simulink model "Simulacion5_1_6_A"  (R2020a)
settings: Solver=VariableStepAuto  StartTime=0.0  StopTime=10.0  RelTol=1e-3
values from neighbouring files (symbols this model uses):
  alpha_cu = 3.9e-3    (= 0.0039)    [AnalisisDeEstabilidad.m]    (also in LTI_vs_LPV_vs_NL_realimentado.m; Modelo_linealizado.m; parametros.m)
  b_eq = b_m + b_l/(r^2)    (= 2.19444444444e-05)    [LTI_vs_LPV_vs_NL_realimentado.m]    (also in Modelo_linealizado.m; parametros.m)
  C_ts = 0.818    [LTI_vs_LPV_vs_NL_realimentado.m]    (also in Modelo_linealizado.m; parametros.m)
  J_eq = J_m + J_l/(r^2)    (= 1.97847222222e-05)    [LTI_vs_LPV_vs_NL_realimentado.m]    (also in Modelo_linealizado.m; parametros.m)
  L_d = 6.6/1000    (= 0.0066)    [Curvas_carc.m]    (also in LTI_vs_LPV_vs_NL_realimentado.m; Modelo_linealizado.m; parametros.m)
  L_ls = 0.8/1000    (= 0.0008)    [LTI_vs_LPV_vs_NL_realimentado.m]    (also in Modelo_linealizado.m; parametros.m)
  L_q = 5.8/1000    (= 0.0058)    [Curvas_carc.m]    (also in LTI_vs_LPV_vs_NL_realimentado.m; Modelo_linealizado.m; parametros.m)
  lambda_m = 0.01546    [Curvas_carc.m]    (also in LTI_vs_LPV_vs_NL_realimentado.m = 0.016; Modelo_linealizado.m = 0.016; parametros.m)
  P_p = 3    [Curvas_carc.m]    (also in LTI_vs_LPV_vs_NL_realimentado.m; parametros.m)
  Pp = 3    [AnalisisDeEstabilidad.m]    (also in LTI_vs_LPV_vs_NL_realimentado.m; Modelo_linealizado.m; parametros.m)
  r = 120    [AnalisisDeEstabilidad.m]    (also in LTI_vs_LPV_vs_NL_realimentado.m; Modelo_linealizado.m; parametros.m)
  R_s = 1.02    [Curvas_carc.m]    (also in LTI_vs_LPV_vs_NL_realimentado.m = R_s_o; Modelo_linealizado.m = 0.348; parametros.m)
  R_sREF = R_sref    (= 1.02)    [LTI_vs_LPV_vs_NL_realimentado.m]    (also in parametros.m)
  R_ts_amb = 146.7    [LTI_vs_LPV_vs_NL_realimentado.m]    (also in Modelo_linealizado.m; parametros.m)
  T_sREF = T_sref    (= 40)    [LTI_vs_LPV_vs_NL_realimentado.m]    (also in parametros.m)
undefined symbols (not defined in the file or in its folder): K_l
libraries: simulink x2
settings Model: Creator=matie  LastModifiedBy=matie

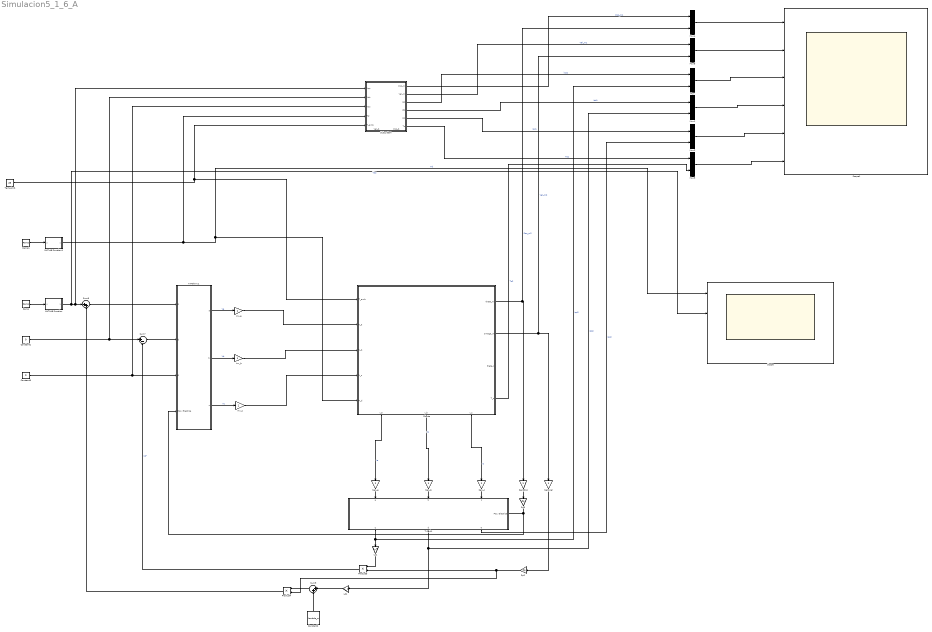
== system Simulacion5_1_6_A ==
  Constant1 : Constant  Value=0
  Constant2 : Constant  Value=lambda_m
  Constant3 : Constant  Value=0
  Inv_a : Gain
  Inv_b : Gain
  Inv_c : Gain
  Ld1 : Gain  Gain=L_d
  Lq1 : Gain  Gain=L_q
  MATLAB Function : MATLAB Function  TreatAsAtomicUnit=on
  MATLAB Function1 : MATLAB Function  TreatAsAtomicUnit=on
  Mux{,1..5} (6 alike) : Mux  Inputs=2
  Planta : Subsystem
      settings: PortSchema="{\"entries\":[{\"content\":{\"sides\":[{\"content\":{\"connectorIds\":[\"In1\",\"In2\",\"In3\",\"In4\",\"In5\"]},\"type\":\"ConnectorPlacement.EquallySpacedRectSide\",\"uuid\":\"7dd159b7-6d73-44ef-8a17-1619ab3a0fe8\"},{\"content\":{\"connectorIds\":[\"Out1\",\"Out2\",\"Out3\",\"Out4\"],\"side\":\"RIGHT\"},\"type\":\"ConnectorPlacement.EquallySpacedRectSide\",\"uuid\":\"f05f5aa2-2d36-48ca-b041-91fd4aa476a9\"},{\"content\":{\"connectorIds\":[],\"side\":\"TOP\"},\"type\":\"ConnectorPlacement.EquallySpacedRectSide\",\"uuid\":\"f00a682c-ef39-4c36-94cc-25936eb5c6a2\"},{\"content\":{\"connectorIds\":[\"Out5\",\"Out6\",\"Out7\"],\"side\":\"BOTTOM\"},\"type\":\"ConnectorPlacement.EquallySpacedRectSide\",\"uuid\":\"801a9ef0-d698-4696-ba24-5671b76f5cda\"}]},\"type\":\"ConnectorPlacement.EquallySpacedConnector\",\"uuid\":\"0722cfee-bb25-4366-9e08-c5916c966df5\"}],\"packageUris\":[\"http://schema.mathworks.com/mf0/Connector/19700101\"],\"version\":\"1.0\"}"
  Pp2 : Gain  Gain=Pp
  Pp3 : Gain  Gain=Pp
  Product3 : Product
  Product4 : Product
  Ramp : simulink/Sources/Ramp  slope=0  start=0  InitialOutput=0
  Ramp1 : simulink/Sources/Ramp  slope=1  start=0  InitialOutput=0
  Scope : Scope  NumInputPorts=4
  Scope1 : Scope  NumInputPorts=6
  Sen_Pos : Gain
  Sen_Vel : Gain
  Sen_a : Gain
  Sen_b : Gain
  Sen_c : Gain
  Subsystem : Subsystem
      settings: PortSchema="{\"entries\":[{\"content\":{\"sides\":[{\"content\":{\"connectorIds\":[\"In1\",\"In2\",\"In3\",\"In4\",\"In5\"]},\"type\":\"ConnectorPlacement.EquallySpacedRectSide\",\"uuid\":\"1d83102d-0bcd-437b-8c43-751b3339846b\"},{\"content\":{\"connectorIds\":[\"Out1\",\"Out2\",\"Out3\",\"Out4\",\"Out5\",\"Out6\"],\"side\":\"RIGHT\"},\"type\":\"ConnectorPlacement.EquallySpacedRectSide\",\"uuid\":\"75e93490-b52d-42b2-adb4-6c409fad0629\"},{\"content\":{\"connectorIds\":[],\"side\":\"TOP\"},\"type\":\"ConnectorPlacement.EquallySpacedRectSide\",\"uuid\":\"c21b1b05-3e78-438e-b61b-25f78d494297\"},{\"content\":{\"connectorIds\":[\"Out7\",\"Out8\"],\"side\":\"BOTTOM\"},\"type\":\"ConnectorPlacement.EquallySpacedRectSide\",\"uuid\":\"0978c98c-ad25-4e7d-b60c-0ad44d3b046e\"}]},\"type\":\"ConnectorPlacement.EquallySpacedConnector\",\"uuid\":\"d07407f3-9cdd-4509-bc17-68fd0115d69d\"}],\"packageUris\":[\"http://schema.mathworks.com/mf0/Connector/19700101\"],\"version\":\"1.0\"}"
  Sum7 : Sum  Inputs=|+-
  Sum8 : Sum  Inputs=|++
  Sum9 : Sum  Inputs=|++
  T.Park1 : Subsystem
      settings: PortSchema="{\"entries\":[{\"content\":{\"sides\":[{\"content\":{\"connectorIds\":[\"In1\",\"In2\",\"In3\"]},\"type\":\"ConnectorPlacement.EquallySpacedRectSide\",\"uuid\":\"2bfbe7ef-652a-4797-b13c-b84c243bd68c\"},{\"content\":{\"connectorIds\":[\"Out1\",\"Out2\",\"Out3\"],\"side\":\"RIGHT\"},\"type\":\"ConnectorPlacement.EquallySpacedRectSide\",\"uuid\":\"075def0e-c436-44dc-ba25-82cf6ffae869\"},{\"content\":{\"connectorIds\":[],\"side\":\"TOP\"},\"type\":\"ConnectorPlacement.EquallySpacedRectSide\",\"uuid\":\"95d81334-e332-4f04-a2cb-c4692f91809c\"},{\"content\":{\"connectorIds\":[\"In4\"],\"side\":\"BOTTOM\"},\"type\":\"ConnectorPlacement.EquallySpacedRectSide\",\"uuid\":\"85b95360-e43d-49d1-a18f-690334b045e6\"}]},\"type\":\"ConnectorPlacement.EquallySpacedConnector\",\"uuid\":\"b90f9cad-0277-459c-bcac-17172872a787\"}],\"packageUris\":[\"http://schema.mathworks.com/mf0/Connector/19700101\"],\"version\":\"1.0\"}"
  T.ParkInv1 : Subsystem
  TempAmb : Constant  Value=25
  wires:
  Constant3/1 -> Subsystem/3(Vos), T.ParkInv1/3(0)
  Sen_c/1 -> T.Park1/3(c)
  Constant1/1 -> Subsystem/2(Vds), Sum7/1
  Sum7/1 -> T.ParkInv1/2(d)
  T.ParkInv1/1(a) -> Inv_a/1  "Va"
  MATLAB Function/1(y) -> Scope/2, Subsystem/1(Vqs), Sum8/1  "Vqs"
  T.ParkInv1/2(b) -> Inv_b/1  "Vb"
  T.ParkInv1/3(c) -> Inv_c/1  "Vc"
  Ramp/1 -> MATLAB Function/1(u)
  Ramp1/1 -> MATLAB Function1/1(u)
  Sum8/1 -> T.ParkInv1/1(q)
  Sum9/1 -> Product4/1
  Product4/1 -> Sum8/2
  Sen_a/1 -> T.Park1/1(a)
  T.Park1/2(d) -> Mux1/2, Ld1/1  "ids2"
  Ld1/1 -> Sum9/1
  T.Park1/1(q) -> Lq1/1, Mux/2  "iqs2"
  Constant2/1 -> Sum9/2
  Sen_Pos/1 -> Pp3/1
  Planta/6(I_b) -> Sen_b/1  "Ib"
  Inv_c/1 -> Planta/4(V_c)
  Sen_b/1 -> T.Park1/2(b)
  MATLAB Function1/1(y) -> Subsystem/4(Td), Planta/5(T_d), Scope/1  "Td"
  Inv_a/1 -> Planta/2(V_a)
  Pp2/1 -> Product4/2, Product3/2
  Planta/5(I_a) -> Sen_a/1  "Ia"
  Sen_Vel/1 -> Pp2/1
  Planta/7(I_c) -> Sen_c/1  "Ic"
  Inv_b/1 -> Planta/3(V_b)
  TempAmb/1 -> Planta/1(T_amb), Subsystem/5(T_amb)
  Pp3/1 -> T.ParkInv1/4(Pos. Electrica), T.Park1/4(Pos. Electrica)
  Lq1/1 -> Product3/1
  Product3/1 -> Sum7/2  "Vd*"
  Subsystem/1(Pos_m) -> Mux4/1  "Pos_m1"
  Subsystem/2(Vel_m) -> Mux5/1  "Vel_m1"
  Subsystem/3(iqs) -> Mux/1  "iqs1"
  Subsystem/4(ids) -> Mux1/1  "ids1"
  Subsystem/5(ios) -> Mux2/1  "ios1"
  Subsystem/6(Ts) -> Mux3/1  "Ts1"
  Planta/2(omega_m) -> Mux5/2, Sen_Vel/1  "Vel_m2"
  Planta/1(theta_m) -> Mux4/2, Sen_Pos/1  "Pos_m2"
  T.Park1/3(0) -> Mux2/2  "ios2"
  Planta/4(T_s) -> Mux3/2  "Ts2"
  Mux4/1 -> Scope1/1
  Mux5/1 -> Scope1/2
  Mux/1 -> Scope1/3
  Mux1/1 -> Scope1/4
  Mux2/1 -> Scope1/5
  Mux3/1 -> Scope1/6

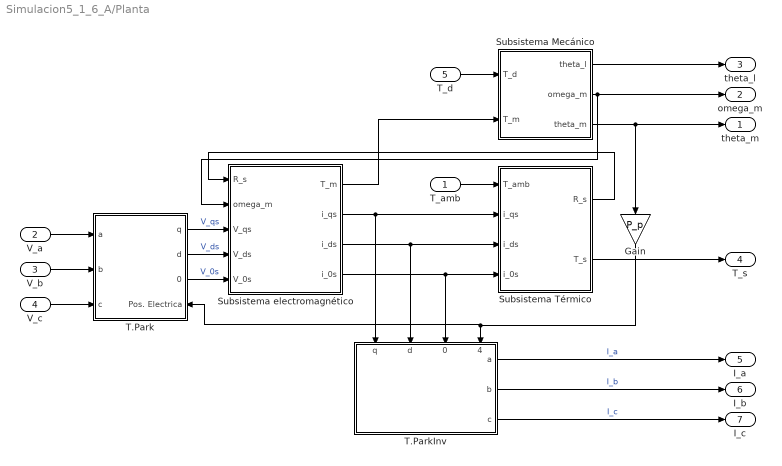
== system Simulacion5_1_6_A/Planta ==
  T_amb : Inport
  V_a : Inport  Port=2
  V_b : Inport  Port=3
  V_c : Inport  Port=4
  T_d : Inport  Port=5
  "\tSubsistema Térmico" : Subsystem
  Gain : Gain  Gain=P_p
  Subsistema Mecánico : Subsystem
  Subsistema electromagnético : Subsystem
  T.Park : Subsystem
      settings: PortSchema="{\"entries\":[{\"content\":{\"sides\":[{\"content\":{\"connectorIds\":[\"In1\",\"In2\",\"In3\"]},\"type\":\"ConnectorPlacement.EquallySpacedRectSide\",\"uuid\":\"2bfbe7ef-652a-4797-b13c-b84c243bd68c\"},{\"content\":{\"connectorIds\":[\"Out1\",\"Out2\",\"Out3\",\"In4\"],\"side\":\"RIGHT\"},\"type\":\"ConnectorPlacement.EquallySpacedRectSide\",\"uuid\":\"075def0e-c436-44dc-ba25-82cf6ffae869\"},{\"content\":{\"connectorIds\":[],\"side\":\"TOP\"},\"type\":\"ConnectorPlacement.EquallySpacedRectSide\",\"uuid\":\"95d81334-e332-4f04-a2cb-c4692f91809c\"}]},\"type\":\"ConnectorPlacement.EquallySpacedConnector\",\"uuid\":\"b90f9cad-0277-459c-bcac-17172872a787\"}],\"packageUris\":[\"http://schema.mathworks.com/mf0/Connector/19700101\"],\"version\":\"1.0\"}"
  T.ParkInv : Subsystem
      settings: PortSchema="{\"entries\":[{\"content\":{\"sides\":[{\"content\":{\"connectorIds\":[\"In1\",\"In2\",\"In3\",\"In4\"]},\"type\":\"ConnectorPlacement.EquallySpacedRectSide\",\"uuid\":\"aef3590a-5fc0-4a95-8f41-1fc79c0f3fe7\"},{\"content\":{\"connectorIds\":[],\"side\":\"RIGHT\"},\"type\":\"ConnectorPlacement.EquallySpacedRectSide\",\"uuid\":\"4e7c387b-9bca-48cc-a151-2357bd6b7b1d\"},{\"content\":{\"connectorIds\":[],\"side\":\"TOP\"},\"type\":\"ConnectorPlacement.EquallySpacedRectSide\",\"uuid\":\"1231932f-f9d3-49e6-b404-2af91cb220c6\"},{\"content\":{\"connectorIds\":[\"Out1\",\"Out2\",\"Out3\"],\"side\":\"BOTTOM\"},\"type\":\"ConnectorPlacement.EquallySpacedRectSide\",\"uuid\":\"4f29e626-7677-496e-bb82-59a3ecbc7a95\"}]},\"type\":\"ConnectorPlacement.EquallySpacedConnector\",\"uuid\":\"48e39a78-817d-4753-b518-4d689d2c1635\"}],\"packageUris\":[\"http://schema.mathworks.com/mf0/Connector/19700101\"],\"version\":\"1.0\"}"
  theta_m : Outport
  omega_m : Outport  Port=2
  theta_l : Outport  Port=3
  T_s : Outport  Port=4
  I_a : Outport  Port=5
  I_b : Outport  Port=6
  I_c : Outport  Port=7
  wires:
  Subsistema Mecánico/3(theta_m) -> Gain/1, theta_m/1
  Gain/1 -> T.Park/4(Pos. Electrica), T.ParkInv/4(Pos. Electrica)
  T.Park/1(q) -> Subsistema electromagnético/3(V_qs)  "V_qs"
  Subsistema Mecánico/2(omega_m) -> Subsistema electromagnético/2(omega_m), omega_m/1
  Subsistema electromagnético/2(i_qs) -> "\tSubsistema Térmico"/2(i_qs), T.ParkInv/1(q)
  Subsistema electromagnético/1(T_m) -> Subsistema Mecánico/2(T_m)
  Subsistema electromagnético/4(i_0s) -> "\tSubsistema Térmico"/4(i_0s), T.ParkInv/3(0)
  V_c/1 -> T.Park/3(c)
  T.ParkInv/3(c) -> I_c/1  "I_c"
  T.ParkInv/2(b) -> I_b/1  "I_b"
  Subsistema electromagnético/3(i_ds) -> "\tSubsistema Térmico"/3(i_ds), T.ParkInv/2(d)
  V_b/1 -> T.Park/2(b)
  Subsistema Mecánico/1(theta_l) -> theta_l/1
  T.ParkInv/1(a) -> I_a/1  "I_a"
  T.Park/3(0) -> Subsistema electromagnético/5(V_0s)  "V_0s"
  V_a/1 -> T.Park/1(a)
  T.Park/2(d) -> Subsistema electromagnético/4(V_ds)  "V_ds"
  T_d/1 -> Subsistema Mecánico/1(T_d)
  T_amb/1 -> "\tSubsistema Térmico"/1(T_amb)
  "\tSubsistema Térmico"/1(R_s) -> Subsistema electromagnético/1(R_s)
  "\tSubsistema Térmico"/2(T_s) -> T_s/1

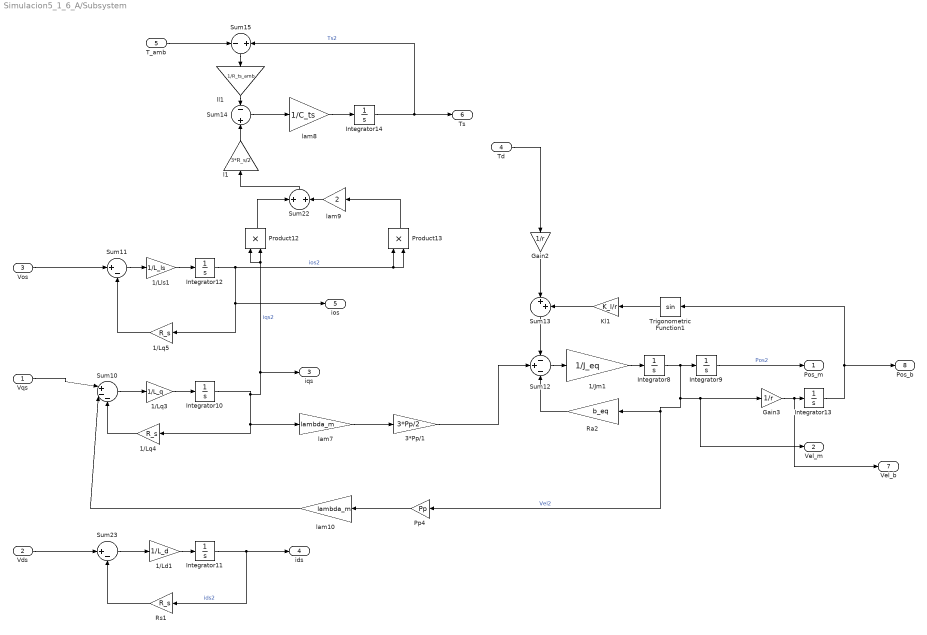
== system Simulacion5_1_6_A/Subsystem ==
  Vqs : Inport
  Vds : Inport  Port=2
  Vos : Inport  Port=3
  Td : Inport  Port=4
  T_amb : Inport  Port=5
  1/Jm1 : Gain  Gain=1/J_eq
  1/Ld1 : Gain  Gain=1/L_d
  1/Lls1 : Gain  Gain=1/L_ls
  1/Lq3 : Gain  Gain=1/L_q
  1/Lq4 : Gain  Gain=R_s
  1/Lq5 : Gain  Gain=R_s
  3*Pp/1 : Gain  Gain=3*Pp/2
  Gain2 : Gain  Gain=1/r
  Gain3 : Gain  Gain=1/r
  Integrator{8..14} (7 alike) : Integrator
  Kl1 : Gain  Gain=K_l/r
  Pp4 : Gain  Gain=Pp
  Product12 : Product
  Product13 : Product
  Ra2 : Gain  Gain=b_eq
  Rs1 : Gain  Gain=R_s
  Sum10 : Sum  Inputs=|+--
  Sum11 : Sum  Inputs=|+-
  Sum12 : Sum  Inputs=-+-
  Sum13 : Sum  Inputs=|++
  Sum14 : Sum  Inputs=-+
  Sum15 : Sum  Inputs=-+
  Sum22 : Sum
  Sum23 : Sum  Inputs=|+-
  Trigonometric Function1 : Trigonometry
  l1 : Gain  Gain=3*R_s/2
  lam10 : Gain  Gain=lambda_m
  lam7 : Gain  Gain=lambda_m
  lam8 : Gain  Gain=1/C_ts
  lam9 : Gain  Gain=2
  ll1 : Gain  Gain=1/R_ts_amb
  Pos_m : Outport
  Vel_m : Outport  Port=2
  iqs : Outport  Port=3
  ids : Outport  Port=4
  ios : Outport  Port=5
  Ts : Outport  Port=6
  Vel_b : Outport  Port=7
  Pos_b : Outport  Port=8
  wires:
  lam9/1 -> Sum22/2
  Vds/1 -> Sum23/1
  1/Jm1/1 -> Integrator8/1
  Integrator11/1 -> ids/1, Rs1/1  "ids2"
  3*Pp/1/1 -> Sum12/2
  Integrator8/1 -> Vel_m/1, Gain3/1, Pp4/1, Ra2/1, Integrator9/1  "Vel2"
  Gain2/1 -> Sum13/1
  Vos/1 -> Sum11/1
  Integrator10/1 -> 1/Lq4/1, lam7/1, iqs/1, Product12/1, Product12/2  "iqs2"
  Product13/1 -> lam9/1
  Pp4/1 -> lam10/1
  Integrator13/1 -> Pos_b/1, Trigonometric Function1/1
  1/Ld1/1 -> Integrator11/1
  Kl1/1 -> Sum13/2
  Td/1 -> Gain2/1
  Integrator14/1 -> Ts/1, Sum15/2  "Ts2"
  Sum12/1 -> 1/Jm1/1
  T_amb/1 -> Sum15/1
  Rs1/1 -> Sum23/2
  Integrator12/1 -> ios/1, 1/Lq5/1, Product13/2, Product13/1  "ios2"
  Sum10/1 -> 1/Lq3/1
  ll1/1 -> Sum14/1
  Trigonometric Function1/1 -> Kl1/1
  Integrator9/1 -> Pos_m/1  "Pos2"
  1/Lq4/1 -> Sum10/3
  lam8/1 -> Integrator14/1
  Product12/1 -> Sum22/1
  Sum11/1 -> 1/Lls1/1
  1/Lq3/1 -> Integrator10/1
  Sum13/1 -> Sum12/1
  lam7/1 -> 3*Pp/1/1
  Sum23/1 -> 1/Ld1/1
  1/Lls1/1 -> Integrator12/1
  Gain3/1 -> Vel_b/1, Integrator13/1
  Ra2/1 -> Sum12/3
  l1/1 -> Sum14/2
  1/Lq5/1 -> Sum11/2
  lam10/1 -> Sum10/2
  Sum15/1 -> ll1/1
  Sum22/1 -> l1/1
  Sum14/1 -> lam8/1
  Vqs/1 -> Sum10/1

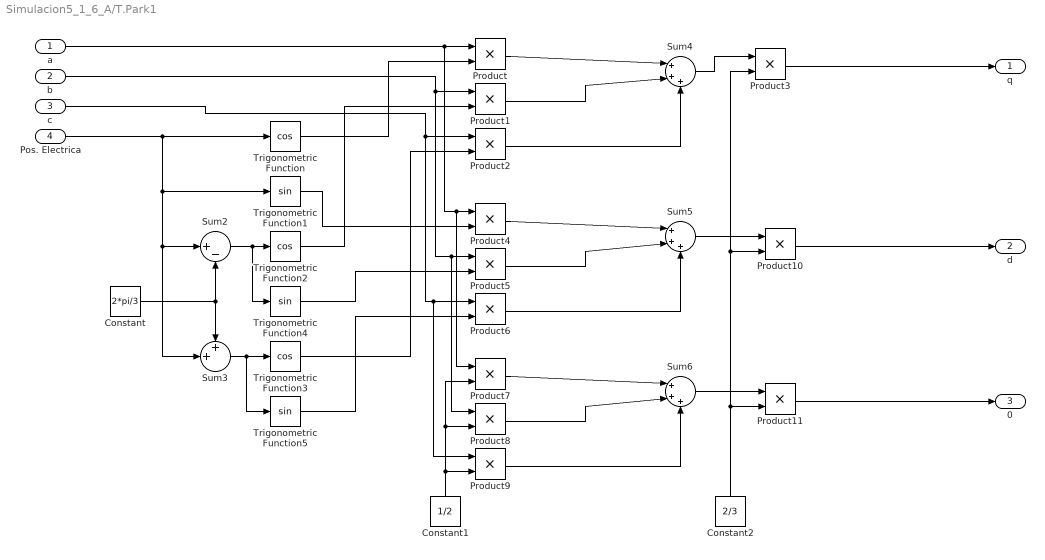
== system Simulacion5_1_6_A/T.Park1 ==
  a : Inport
  b : Inport  Port=2
  c : Inport  Port=3
  Pos. Electrica : Inport  Port=4
  Constant : Constant  Value=2*pi/3
  Constant1 : Constant  Value=1/2
  Constant2 : Constant  Value=2/3
  Product{,1..11} (12 alike) : Product
  Sum2 : Sum  Inputs=|+-
  Sum3 : Sum  Inputs=++|
  Sum4 : Sum  Inputs=|+++
  Sum5 : Sum  Inputs=|+++
  Sum6 : Sum  Inputs=|+++
  Trigonometric Function : Trigonometry  Operator=cos
  Trigonometric Function1 : Trigonometry
  Trigonometric Function2 : Trigonometry  Operator=cos
  Trigonometric Function3 : Trigonometry  Operator=cos
  Trigonometric Function4 : Trigonometry
  Trigonometric Function5 : Trigonometry
  q : Outport
  d : Outport  Port=2
  0 : Outport  Port=3
  wires:
  Product1/1 -> Sum4/2
  c/1 -> Product9/1, Product6/1, Product2/1
  Constant1/1 -> Product9/2, Product8/2, Product7/2
  Sum2/1 -> Trigonometric Function4/1, Trigonometric Function2/1
  Constant2/1 -> Product11/2, Product10/2, Product3/2
  b/1 -> Product8/1, Product5/1, Product1/1
  Product11/1 -> 0/1
  Pos. Electrica/1 -> Sum3/2, Sum2/1, Trigonometric Function1/1, Trigonometric Function/1
  Trigonometric Function2/1 -> Product1/2
  Trigonometric Function5/1 -> Product6/2
  Product6/1 -> Sum5/3
  Trigonometric Function1/1 -> Product4/2
  Constant/1 -> Sum3/1, Sum2/2
  Sum5/1 -> Product10/1
  Product3/1 -> q/1
  Sum4/1 -> Product3/1
  Trigonometric Function3/1 -> Product2/2
  Trigonometric Function/1 -> Product/2
  a/1 -> Product7/1, Product4/1, Product/1
  Product10/1 -> d/1
  Trigonometric Function4/1 -> Product5/2
  Product/1 -> Sum4/1
  Product7/1 -> Sum6/1
  Sum3/1 -> Trigonometric Function5/1, Trigonometric Function3/1
  Product2/1 -> Sum4/3
  Product9/1 -> Sum6/3
  Product5/1 -> Sum5/2
  Product4/1 -> Sum5/1
  Sum6/1 -> Product11/1
  Product8/1 -> Sum6/2

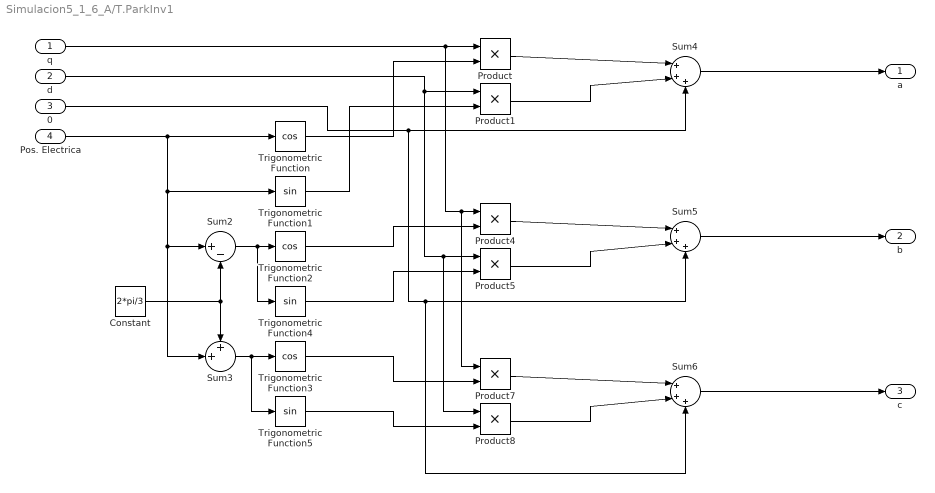
== system Simulacion5_1_6_A/T.ParkInv1 ==
  q : Inport
  d : Inport  Port=2
  0 : Inport  Port=3
  Pos. Electrica : Inport  Port=4
  Constant : Constant  Value=2*pi/3
  Product{,1,4..5,7..8} (6 alike) : Product
  Sum2 : Sum  Inputs=|+-
  Sum3 : Sum  Inputs=++|
  Sum4 : Sum  Inputs=|+++
  Sum5 : Sum  Inputs=|+++
  Sum6 : Sum  Inputs=|+++
  Trigonometric Function : Trigonometry  Operator=cos
  Trigonometric Function1 : Trigonometry
  Trigonometric Function2 : Trigonometry  Operator=cos
  Trigonometric Function3 : Trigonometry  Operator=cos
  Trigonometric Function4 : Trigonometry
  Trigonometric Function5 : Trigonometry
  a : Outport
  b : Outport  Port=2
  c : Outport  Port=3
  wires:
  Constant/1 -> Sum3/1, Sum2/2
  Pos. Electrica/1 -> Sum3/2, Sum2/1, Trigonometric Function1/1, Trigonometric Function/1
  Trigonometric Function3/1 -> Product7/2
  d/1 -> Product8/1, Product5/1, Product1/1
  0/1 -> Sum4/3, Sum5/3, Sum6/3
  Product8/1 -> Sum6/2
  Product7/1 -> Sum6/1
  q/1 -> Product7/1, Product4/1, Product/1
  Sum3/1 -> Trigonometric Function5/1, Trigonometric Function3/1
  Trigonometric Function5/1 -> Product8/2
  Sum6/1 -> c/1
  Product1/1 -> Sum4/2
  Sum2/1 -> Trigonometric Function4/1, Trigonometric Function2/1
  Sum4/1 -> a/1
  Sum5/1 -> b/1
  Trigonometric Function1/1 -> Product1/2
  Product5/1 -> Sum5/2
  Trigonometric Function2/1 -> Product4/2
  Product4/1 -> Sum5/1
  Product/1 -> Sum4/1
  Trigonometric Function/1 -> Product/2
  Trigonometric Function4/1 -> Product5/2

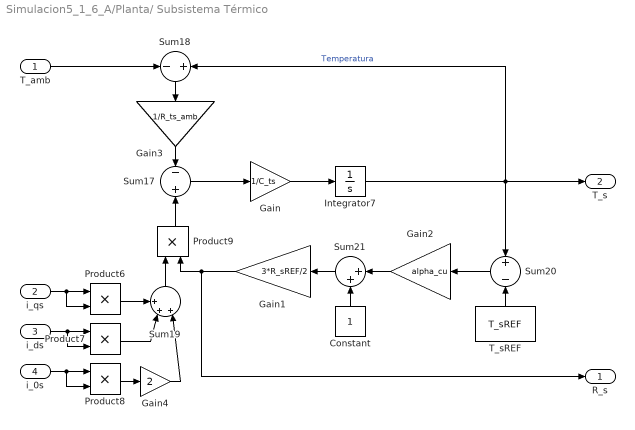
== system Simulacion5_1_6_A/Planta/	Subsistema Térmico ==
  T_amb : Inport
  i_qs : Inport  Port=2
  i_ds : Inport  Port=3
  i_0s : Inport  Port=4
  Constant : Constant
  Gain : Gain  Gain=1/C_ts
  Gain1 : Gain  Gain=3*R_sREF/2
  Gain2 : Gain  Gain=alpha_cu
  Gain3 : Gain  Gain=1/R_ts_amb
  Gain4 : Gain  Gain=2
  Integrator7 : Integrator
  Product{6..9} (4 alike) : Product
  Sum17 : Sum  Inputs=-+
  Sum18 : Sum  Inputs=-+
  Sum19 : Sum  Inputs=+++|
  Sum20 : Sum  Inputs=+-
  Sum21 : Sum  Inputs=|++
  T_sREF : Constant  Value=T_sREF
  R_s : Outport
  T_s : Outport  Port=2
  wires:
  Gain4/1 -> Sum19/3
  Integrator7/1 -> Sum18/2, T_s/1, Sum20/1  "Temperatura"
  Sum21/1 -> Gain1/1
  i_ds/1 -> Product7/2, Product7/1
  Product8/1 -> Gain4/1
  Product7/1 -> Sum19/2
  T_amb/1 -> Sum18/1
  Sum18/1 -> Gain3/1
  Product6/1 -> Sum19/1
  Gain/1 -> Integrator7/1
  Product9/1 -> Sum17/2
  Sum17/1 -> Gain/1
  Gain3/1 -> Sum17/1
  T_sREF/1 -> Sum20/2
  Sum20/1 -> Gain2/1
  Gain1/1 -> Product9/2, R_s/1
  i_qs/1 -> Product6/1, Product6/2
  Sum19/1 -> Product9/1
  Gain2/1 -> Sum21/1
  i_0s/1 -> Product8/2, Product8/1
  Constant/1 -> Sum21/2

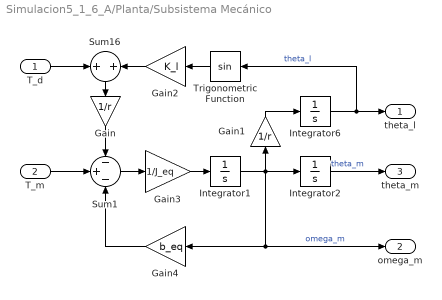
== system Simulacion5_1_6_A/Planta/Subsistema Mecánico ==
  T_d : Inport
  T_m : Inport  Port=2
  Gain : Gain  Gain=1/r
  Gain1 : Gain  Gain=1/r
  Gain2 : Gain  Gain=K_l
  Gain3 : Gain  Gain=1/J_eq
  Gain4 : Gain  Gain=b_eq
  Integrator1 : Integrator
  Integrator2 : Integrator
  Integrator6 : Integrator
  Sum1 : Sum  Inputs=-+-
  Sum16 : Sum  Inputs=+|+
  Trigonometric Function : Trigonometry
  theta_l : Outport
  omega_m : Outport  Port=2
  theta_m : Outport  Port=3
  wires:
  Integrator2/1 -> theta_m/1  "theta_m"
  Integrator6/1 -> theta_l/1, Trigonometric Function/1  "theta_l"
  Gain1/1 -> Integrator6/1
  Gain4/1 -> Sum1/3
  T_m/1 -> Sum1/2
  Integrator1/1 -> Gain4/1, omega_m/1, Integrator2/1, Gain1/1  "omega_m"
  Trigonometric Function/1 -> Gain2/1
  Gain2/1 -> Sum16/2
  Sum16/1 -> Gain/1
  Gain/1 -> Sum1/1
  T_d/1 -> Sum16/1
  Sum1/1 -> Gain3/1
  Gain3/1 -> Integrator1/1

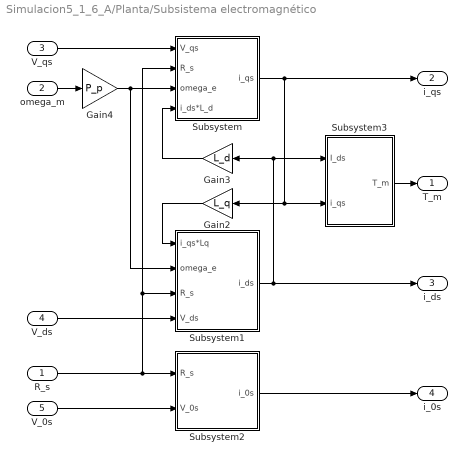
== system Simulacion5_1_6_A/Planta/Subsistema electromagnético ==
  R_s : Inport
  omega_m : Inport  Port=2
  V_qs : Inport  Port=3
  V_ds : Inport  Port=4
  V_0s : Inport  Port=5
  Gain2 : Gain  Gain=L_q
  Gain3 : Gain  Gain=L_d
  Gain4 : Gain  Gain=P_p
  Subsystem : Subsystem
  Subsystem1 : Subsystem
  Subsystem2 : Subsystem
  Subsystem3 : Subsystem
  T_m : Outport
  i_qs : Outport  Port=2
  i_ds : Outport  Port=3
  i_0s : Outport  Port=4
  wires:
  omega_m/1 -> Gain4/1
  Subsystem/1(i_qs) -> i_qs/1, Subsystem3/2(i_qs), Gain2/1
  Subsystem1/1(i_ds) -> i_ds/1, Subsystem3/1(I_ds), Gain3/1
  Gain2/1 -> Subsystem1/1(i_qs*Lq)
  Gain3/1 -> Subsystem/4(i_ds*L_d)
  Gain4/1 -> Subsystem1/2(omega_e), Subsystem/3(omega_e)
  V_qs/1 -> Subsystem/1(V_qs)
  R_s/1 -> Subsystem/2(R_s), Subsystem1/3(R_s), Subsystem2/1(R_s)
  V_ds/1 -> Subsystem1/4(V_ds)
  V_0s/1 -> Subsystem2/2(V_0s)
  Subsystem2/1(i_0s) -> i_0s/1
  Subsystem3/1(T_m) -> T_m/1

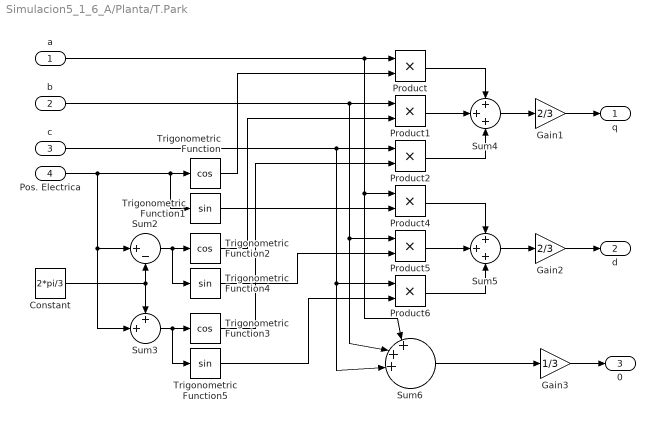
== system Simulacion5_1_6_A/Planta/T.Park ==
  a : Inport
  b : Inport  Port=2
  c : Inport  Port=3
  Pos. Electrica : Inport  Port=4
  Constant : Constant  Value=2*pi/3
  Gain1 : Gain  Gain=2/3
  Gain2 : Gain  Gain=2/3
  Gain3 : Gain  Gain=1/3
  Product{,1..2,4..6} (6 alike) : Product
  Sum2 : Sum  Inputs=|+-
  Sum3 : Sum  Inputs=++|
  Sum4 : Sum  Inputs=+++
  Sum5 : Sum  Inputs=+++
  Sum6 : Sum  Inputs=|+|+|+||||
  Trigonometric Function : Trigonometry  Operator=cos
  Trigonometric Function1 : Trigonometry
  Trigonometric Function2 : Trigonometry  Operator=cos
  Trigonometric Function3 : Trigonometry  Operator=cos
  Trigonometric Function4 : Trigonometry
  Trigonometric Function5 : Trigonometry
  q : Outport
  d : Outport  Port=2
  0 : Outport  Port=3
  wires:
  Product1/1 -> Sum4/2
  c/1 -> Product2/1, Product6/1, Sum6/3
  Sum2/1 -> Trigonometric Function4/1, Trigonometric Function2/1
  b/1 -> Product1/1, Product5/1, Sum6/2
  Pos. Electrica/1 -> Trigonometric Function/1, Trigonometric Function1/1, Sum3/2, Sum2/1
  Trigonometric Function2/1 -> Product1/2
  Trigonometric Function5/1 -> Product6/2
  Product6/1 -> Sum5/3
  Trigonometric Function1/1 -> Product4/2
  Constant/1 -> Sum3/1, Sum2/2
  Sum5/1 -> Gain2/1
  Gain1/1 -> q/1
  Sum4/1 -> Gain1/1
  Trigonometric Function3/1 -> Product2/2
  Trigonometric Function/1 -> Product/2
  a/1 -> Product4/1, Sum6/1, Product/1
  Trigonometric Function4/1 -> Product5/2
  Product/1 -> Sum4/1
  Sum3/1 -> Trigonometric Function5/1, Trigonometric Function3/1
  Product2/1 -> Sum4/3
  Product5/1 -> Sum5/2
  Product4/1 -> Sum5/1
  Sum6/1 -> Gain3/1
  Gain3/1 -> 0/1
  Gain2/1 -> d/1

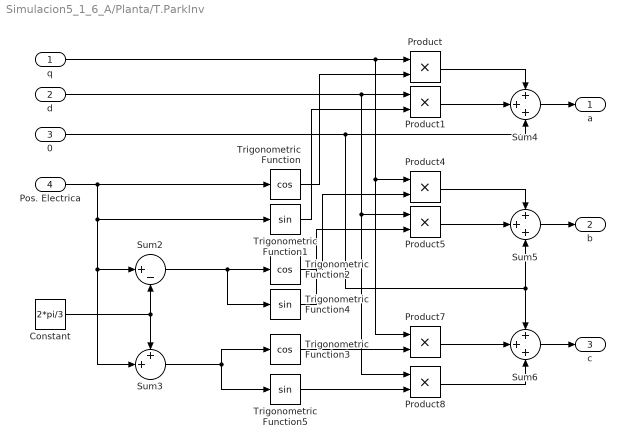
== system Simulacion5_1_6_A/Planta/T.ParkInv ==
  q : Inport
  d : Inport  Port=2
  0 : Inport  Port=3
  Pos. Electrica : Inport  Port=4
  Constant : Constant  Value=2*pi/3
  Product{,1,4..5,7..8} (6 alike) : Product
  Sum2 : Sum  Inputs=|+-
  Sum3 : Sum  Inputs=++|
  Sum4 : Sum  Inputs=+++
  Sum5 : Sum  Inputs=+++
  Sum6 : Sum  Inputs=+++
  Trigonometric Function : Trigonometry  Operator=cos
  Trigonometric Function1 : Trigonometry
  Trigonometric Function2 : Trigonometry  Operator=cos
  Trigonometric Function3 : Trigonometry  Operator=cos
  Trigonometric Function4 : Trigonometry
  Trigonometric Function5 : Trigonometry
  a : Outport
  b : Outport  Port=2
  c : Outport  Port=3
  wires:
  Constant/1 -> Sum3/1, Sum2/2
  Pos. Electrica/1 -> Sum3/2, Sum2/1, Trigonometric Function1/1, Trigonometric Function/1
  Trigonometric Function3/1 -> Product7/2
  d/1 -> Product8/1, Product5/1, Product1/1
  0/1 -> Sum6/1, Sum5/3, Sum4/3
  Product8/1 -> Sum6/3
  Product7/1 -> Sum6/2
  q/1 -> Product7/1, Product4/1, Product/1
  Sum3/1 -> Trigonometric Function5/1, Trigonometric Function3/1
  Trigonometric Function5/1 -> Product8/2
  Sum6/1 -> c/1
  Product1/1 -> Sum4/2
  Sum2/1 -> Trigonometric Function4/1, Trigonometric Function2/1
  Sum4/1 -> a/1
  Sum5/1 -> b/1
  Trigonometric Function1/1 -> Product1/2
  Product5/1 -> Sum5/2
  Trigonometric Function2/1 -> Product4/2
  Product4/1 -> Sum5/1
  Product/1 -> Sum4/1
  Trigonometric Function/1 -> Product/2
  Trigonometric Function4/1 -> Product5/2

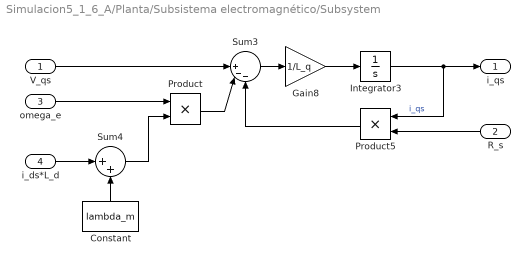
== system Simulacion5_1_6_A/Planta/Subsistema electromagnético/Subsystem ==
  V_qs : Inport
  R_s : Inport  Port=2
  omega_e : Inport  Port=3
  i_ds*L_d : Inport  Port=4
  Constant : Constant  Value=lambda_m
  Gain8 : Gain  Gain=1/L_q
  Integrator3 : Integrator
  Product : Product
  Product5 : Product
  Sum3 : Sum  Inputs=||+--
  Sum4 : Sum  Inputs=|++
  i_qs : Outport
  wires:
  Constant/1 -> Sum4/2
  Product5/1 -> Sum3/3
  V_qs/1 -> Sum3/1
  i_ds*L_d/1 -> Sum4/1
  Product/1 -> Sum3/2
  Gain8/1 -> Integrator3/1
  Integrator3/1 -> Product5/1, i_qs/1  "i_qs"
  Sum4/1 -> Product/2
  Sum3/1 -> Gain8/1
  R_s/1 -> Product5/2
  omega_e/1 -> Product/1

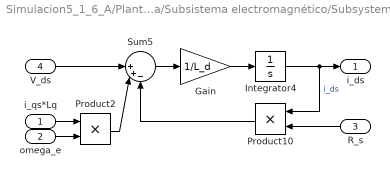
== system Simulacion5_1_6_A/Planta/Subsistema electromagnético/Subsystem1 ==
  i_qs*Lq : Inport
  omega_e : Inport  Port=2
  R_s : Inport  Port=3
  V_ds : Inport  Port=4
  Gain : Gain  Gain=1/L_d
  Integrator4 : Integrator
  Product10 : Product
  Product2 : Product
  Sum5 : Sum  Inputs=||++-
  i_ds : Outport
  wires:
  Product10/1 -> Sum5/3
  i_qs*Lq/1 -> Product2/1
  Gain/1 -> Integrator4/1
  V_ds/1 -> Sum5/1
  Sum5/1 -> Gain/1
  R_s/1 -> Product10/2
  Product2/1 -> Sum5/2
  omega_e/1 -> Product2/2
  Integrator4/1 -> i_ds/1, Product10/1  "i_ds"

== system Simulacion5_1_6_A/Planta/Subsistema electromagnético/Subsystem2 ==
  R_s : Inport
  V_0s : Inport  Port=2
  Gain1 : Gain  Gain=1/L_ls
  Integrator5 : Integrator
  Product11 : Product
  Sum6 : Sum  Inputs=|+-
  i_0s : Outport
  wires:
  Integrator5/1 -> i_0s/1, Product11/1  "i_0s"
  Product11/1 -> Sum6/2
  R_s/1 -> Product11/2
  Sum6/1 -> Gain1/1
  Gain1/1 -> Integrator5/1
  V_0s/1 -> Sum6/1

== system Simulacion5_1_6_A/Planta/Subsistema electromagnético/Subsystem3 ==
  I_ds : Inport
  i_qs : Inport  Port=2
  Gain5 : Gain  Gain=L_d-L_q
  Gain6 : Gain  Gain=3*P_p/2
  Gain7 : Gain  Gain=lambda_m
  Product1 : Product
  Sum2 : Sum  Inputs=|++
  T_m : Outport
  wires:
  Sum2/1 -> Gain6/1
  Gain7/1 -> Sum2/1
  I_ds/1 -> Product1/2
  Gain5/1 -> Sum2/2
  i_qs/1 -> Product1/1, Gain7/1
  Gain6/1 -> T_m/1
  Product1/1 -> Gain5/1

== matlab function Simulacion5_1_6_A/MATLAB Function ==
  data: u input; y output
function y = fcn(u)
y = 0;
if (u>=0.1)&&(u<=0.7)
    y = 19.596;
end

== matlab function Simulacion5_1_6_A/MATLAB Function1 ==
  data: u input; y output
function y = fcn(u)
y = 0;
if (u>=0.3)&&(u<=0.5)
    y = 6.28;
end
if (u>0.5)&&(u<=0.9)
    y = -6.28;
end
